simulink model "HSimpleConstDead"  (Simulink 7.9)
settings: Solver=FixedStepDiscrete  StartTime=0.0  StopTime=100000000.0  FixedStep=1  RelTol=1e-3
settings Model: Creator=boakes  LastModifiedBy=boakes
settings OptimizationCC: BlockReduction=off  ConditionallyExecuteInputs=off  EnhancedBackFolding=on

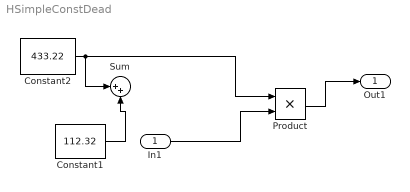
== system HSimpleConstDead ==
  In1 : Inport
  Constant1 : Constant  Value=112.32
  Constant2 : Constant  Value=433.22
  Product : Product  RndMeth=Zero
  Sum : Sum  Inputs=|++
  Out1 : Outport
  wires:
  Constant1/1 -> Sum/2
  In1/1 -> Product/2
  Product/1 -> Out1/1
  Constant2/1 -> Sum/1, Product/1
